simulink model "Simscape_crane_software_model"  (R2016b)
settings: Solver=ode15s  StartTime=0.0  StopTime=3  RelTol=1e-3  EnableMultiTasking=on
values from neighbouring files (symbols this model uses):
  m = 0.47    [SSmodelParams.mat]
  MR = 1.71    [SSmodelParams.mat]
  TxBreak = 0    [setup.m]
  TxCoulomb = 2.5    [setup.m]
  TxVisc = 49.1750    (= 49.175)    [setup.m]
  TyBreak = 0    [setup.m]
  TyCoulomb = 1.8    [setup.m]
  xZero = 0    [setup.m]
  yZero = 0    [setup.m]
undefined symbols (not defined in the file or in its folder): sigbuilder_block, TzBreak, TzCoulomb, X, xRange, Y, yRange, Z, zRange, zZero
undefined symbols (not defined in the file): M, TorqueMultX, TorqueMultY, TorqueMultZ, TxTrans, TyTrans, TyVisc, TzTrans, TzVisc
libraries: sm_lib x146, fl_lib x62, nesl_utility x24, elec_lib x9, simulink x6, sm_double_wishbone_suspension_lib x4, aerolibtransform2 x1
(part 11 of 14)

== system Simscape_crane_software_model/0.4 ==
  Demux : Demux  Tag=STV Demux  Outputs=1
  FromWs : FromWorkspace  Tag=STV FromWs  VariableName=tuvar  SampleTime=0
      SigBuilderData=|
      | common.afterFinalStr = 'Extrapolate'
      | common.sampleTime = 0
      | dataSet.timeRange = [0 10]
      | dataSet.name = 'Group 1'
      | sbobj.Groups.Name = 'Group 1'
      | sbobj.Groups.Signals.Name = 'Signal 1'
      | sbobj.Groups.Signals.XData = [0 1 1 2 2 10]
      | sbobj.Groups.Signals.YData = [0 0 0.4 0.4 0 0]
  Signal 1 : Outport  Tag=STV Outport
  wires:
  Demux/1 -> Signal 1/1
  FromWs/1 -> Demux/1

== system Simscape_crane_software_model/0.8 ==
  Demux : Demux  Tag=STV Demux  Outputs=1
  FromWs : FromWorkspace  Tag=STV FromWs  VariableName=tuvar  SampleTime=0
      SigBuilderData=|
      | common.afterFinalStr = 'Extrapolate'
      | common.sampleTime = 0
      | dataSet.timeRange = [0 10]
      | dataSet.name = 'Group 1'
      | sbobj.Groups.Name = 'Group 1'
      | sbobj.Groups.Signals.Name = 'Signal 1'
      | sbobj.Groups.Signals.XData = [0 1 1 2 2 10]
      | sbobj.Groups.Signals.YData = [0 0 0.8 0.8 0 0]
  Signal 1 : Outport  Tag=STV Outport
  wires:
  FromWs/1 -> Demux/1
  Demux/1 -> Signal 1/1

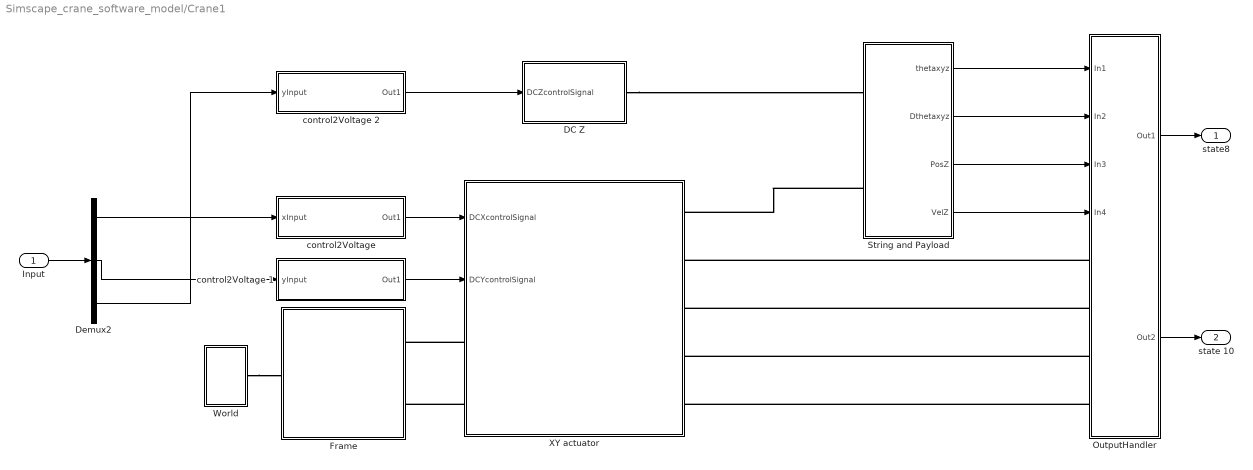
== system Simscape_crane_software_model/Crane1 ==
  Input : Inport
  DC Z : Subsystem
  Demux2 : Demux  Outputs=3
  Frame : Subsystem
  OutputHandler : Subsystem
  String and Payload : Subsystem
  World : Subsystem
  XY actuator : Subsystem
  "control2Voltage " : Subsystem
      mask Display:
      | port_label('output', 1, 'pwm_out')
      | port_label('input', 1, 'controlVal')
  control2Voltage 1 : Subsystem
      mask Display:
      | port_label('output', 1, 'pwm_out')
      | port_label('input', 1, 'controlVal')
  control2Voltage 2 : Subsystem
      mask Display:
      | port_label('output', 1, 'pwm_out')
      | port_label('input', 1, 'controlVal')
  "state8 " : Outport
  state 10 : Outport  Port=2
  wires:
  "control2Voltage "/1(Out1) -> XY actuator/1(DCXcontrolSignal)
  control2Voltage 1/1(Out1) -> XY actuator/2(DCYcontrolSignal)
  Demux2/1 -> "control2Voltage "/1(xInput)
  Demux2/2 -> control2Voltage 1/1(yInput)
  Input/1 -> Demux2/1
  Demux2/3 -> control2Voltage 2/1(yInput)
  control2Voltage 2/1(Out1) -> DC Z/1(DCZcontrolSignal)
  String and Payload/1(thetaxyz) -> OutputHandler/1(In1)
  String and Payload/2(Dthetaxyz) -> OutputHandler/2(In2)
  String and Payload/3("PosZ ") -> OutputHandler/3(In3)
  String and Payload/4(VelZ) -> OutputHandler/4(In4)
  OutputHandler/1(Out1) -> "state8 "/1
  OutputHandler/2(Out2) -> state 10/1
  connections:
  World/RConn1 -- Frame/LConn1
  XY actuator/LConn1 -- Frame/RConn1
  XY actuator/LConn2 -- Frame/RConn2
  String and Payload/LConn2 -- XY actuator/RConn1
  DC Z/RConn1 -- String and Payload/LConn1
  OutputHandler/LConn1 -- XY actuator/RConn2
  OutputHandler/LConn2 -- XY actuator/RConn3
  OutputHandler/LConn3 -- XY actuator/RConn4
  OutputHandler/LConn4 -- XY actuator/RConn5

== system Simscape_crane_software_model/Crane1/DC Z ==
  DCZcontrolSignal : Inport
  " Lead Screw" : fl_lib/Mechanical/Mechanisms/Wheel and Axle  R=6 cm  or=1  t_specify=off  t_priority=High  t=0 N*m  f_specify=off  f_priority=High  f=0 N
  DC Motor2 : elec_lib/Actuators & Drivers/Rotational Actuators/DC Motor  parameterization=2  Ra=3.9 Ohm  La=1.2e-5 H  emf_or_torque=1  Kv=7.2e-5 V/rpm  Ki=6.876e-4 N*m/A  T_stall=10000 mN*m  w_max=190 rpm  w_rated=190 rpm  P_rated=0.08 W  V_rated=24 V  J=0.01 g*cm^2  lam_param=1  lam=0 N*m/(rad/s)  i_noload=0 A  V_i_noload=1.5 V  speed0=0 rpm  alpha=0.00393 1/K  Tmeas=25 C  thermal_mass=100 J/K  initial_temperature=25 C
  Force Sensor : fl_lib/Mechanical/Mechanical Sensors/Ideal Force Sensor
  Gear Box : fl_lib/Mechanical/Mechanisms/Gear Box  Tag=Factory Generic  ratio=1/30  t_in_specify=off  t_in_priority=High  t_in=0 N*m  t_out_specify=off  t_out_priority=High  t_out=0 N*m
  Mechanical Rotational Reference1 : fl_lib/Mechanical/Rotational Elements/Mechanical Rotational Reference
  Mechanical Translational Reference4 : fl_lib/Mechanical/Translational Elements/Mechanical Translational Reference
  PS Gain : fl_lib/Physical Signals/Functions/PS Gain  gain=-Uz
  PWM & H-Bridge1 : Subsystem
  SL2V_1 : Subsystem
  Conn1 : PMIOPort  Port=1  Side=Right
  wires:
  DCZcontrolSignal/1 -> SL2V_1/1(SL)
  connections:
  Force Sensor/RConn2 -- PS Gain/LConn1
  Mechanical Translational Reference4/LConn1 -- Force Sensor/LConn1
  Mechanical Rotational Reference1/LConn1 -- DC Motor2/RConn2
  Gear Box/RConn1 -- " Lead Screw"/LConn1
  Force Sensor/RConn1 -- " Lead Screw"/RConn1
  DC Motor2/LConn2 -- Gear Box/LConn1
  PWM & H-Bridge1/RConn2 -- DC Motor2/RConn1
  SL2V_1/RConn2 -- PWM & H-Bridge1/LConn2
  SL2V_1/RConn3 -- PWM & H-Bridge1/LConn3
  SL2V_1/RConn4 -- PWM & H-Bridge1/LConn4
  SL2V_1/RConn1 -- PWM & H-Bridge1/LConn1
  PWM & H-Bridge1/RConn1 -- DC Motor2/LConn1
  Conn1/RConn1 -- PS Gain/RConn1

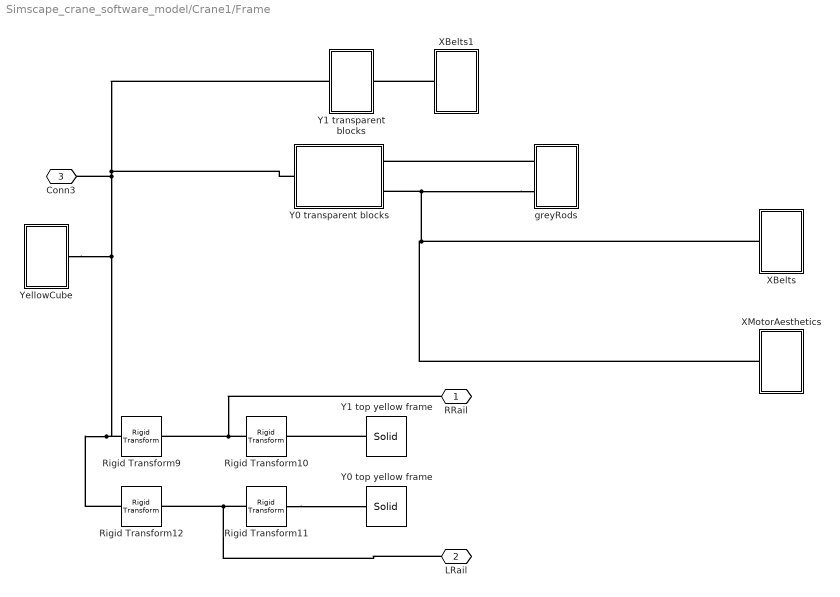
== system Simscape_crane_software_model/Crane1/Frame ==
  Rigid Transform10 : sm_lib/Frames and Transforms/Rigid Transform  TranslationMethod=None  TranslationStandardOffset=0  TranslationLengthUnit=m  TranslationStandardAxis=+Z  TranslationCartesianOffset="[-0.5 1  0]"  TranslationROffset=0  TranslationROffsetUnits=m  TranslationZOffset=0  TranslationZOffsetUnits=m  TranslationThetaOffset=0  TranslationThetaOffsetUnits=deg  RotationMethod=StandardAxis  RotationAngleUnits=deg  RotationStandardAxis=+Y  RotationAngle=90  RotationArbitraryAxis=[0 0 1]  FollAlignAxisA=+X  BaseAlignAxisA=+Y  FollAlignAxisB=+Y  BaseAlignAxisB=+Z  RotationSequenceAxes=FollowerAxes  RotationSequence=XYX  RotationSequenceAngles=[0 0 0]  RotationSequenceAnglesUnits=deg  RotationMatrix=[1 0 0; 0 1 0; 0 0 1]
  Rigid Transform11 : sm_lib/Frames and Transforms/Rigid Transform  TranslationMethod=None  TranslationStandardOffset=0  TranslationLengthUnit=m  TranslationStandardAxis=+Z  TranslationCartesianOffset="[-0.5 1  0]"  TranslationROffset=0  TranslationROffsetUnits=m  TranslationZOffset=0  TranslationZOffsetUnits=m  TranslationThetaOffset=0  TranslationThetaOffsetUnits=deg  RotationMethod=StandardAxis  RotationAngleUnits=deg  RotationStandardAxis=+Y  RotationAngle=90  RotationArbitraryAxis=[0 0 1]  FollAlignAxisA=+X  BaseAlignAxisA=+Y  FollAlignAxisB=+Y  BaseAlignAxisB=+Z  RotationSequenceAxes=FollowerAxes  RotationSequence=XYX  RotationSequenceAngles=[0 0 0]  RotationSequenceAnglesUnits=deg  RotationMatrix=[1 0 0; 0 1 0; 0 0 1]
  Rigid Transform12 : sm_lib/Frames and Transforms/Rigid Transform  TranslationMethod=Cartesian  TranslationStandardOffset=0  TranslationLengthUnit=m  TranslationStandardAxis=+Z  TranslationCartesianOffset=[0 -0.5 1]  TranslationROffset=0  TranslationROffsetUnits=m  TranslationZOffset=0  TranslationZOffsetUnits=m  TranslationThetaOffset=0  TranslationThetaOffsetUnits=deg  RotationMethod=None  RotationAngleUnits=deg  RotationStandardAxis=+X  RotationAngle=90  RotationArbitraryAxis=[0 0 1]  FollAlignAxisA=+X  BaseAlignAxisA=+Y  FollAlignAxisB=+Y  BaseAlignAxisB=+Z  RotationSequenceAxes=FollowerAxes  RotationSequence=XYX  RotationSequenceAngles=[0 0 0]  RotationSequenceAnglesUnits=deg  RotationMatrix=[1 0 0; 0 1 0; 0 0 1]
  Rigid Transform9 : sm_lib/Frames and Transforms/Rigid Transform  TranslationMethod=Cartesian  TranslationStandardOffset=0  TranslationLengthUnit=m  TranslationStandardAxis=+Z  TranslationCartesianOffset=[0 0.5 1]  TranslationROffset=0  TranslationROffsetUnits=m  TranslationZOffset=0  TranslationZOffsetUnits=m  TranslationThetaOffset=0  TranslationThetaOffsetUnits=deg  RotationMethod=None  RotationAngleUnits=deg  RotationStandardAxis=+X  RotationAngle=90  RotationArbitraryAxis=[0 0 1]  FollAlignAxisA=+X  BaseAlignAxisA=+Y  FollAlignAxisB=+Y  BaseAlignAxisB=+Z  RotationSequenceAxes=FollowerAxes  RotationSequence=XYX  RotationSequenceAngles=[0 0 0]  RotationSequenceAnglesUnits=deg  RotationMatrix=[1 0 0; 0 1 0; 0 0 1]
  XBelts : Subsystem
  XBelts1 : Subsystem
  XMotorAesthetics : Subsystem
  Y0 top yellow frame : sm_lib/Body Elements/Solid  InertiaType=CalculateFromGeometry  Mass=1  MassUnits=kg  CenterOfMass=[0 0 0]  CenterOfMassUnits=m  MomentsOfInertia=[1 1 1]  MomentsOfInertiaUnits=kg*m^2  ProductsOfInertia=[0 0 0]  ProductsOfInertiaUnits=kg*m^2  DensityBased=on  Density=1000  DensityUnits=kg/(m^3)  DoExposeReferenceFrame=on  SerializedFrames=<Frames/>  GraphicType=FromGeometry  MarkerShape=Sphere  MarkerSize=10  MarkerSizeUnits=m  GraphicVisPropType=SimpleVisualProperties  GraphicDiffuseColor=[1.0 1.0 0.2]  GraphicSpecularColor=[0.5 0.5 0.5 1.0]  GraphicAmbientColor=[0.15 0.15 0.15 1.0]  GraphicEmissiveColor=[0.0 0.0 0.0 1.0]  GraphicShininess=75  GraphicOpacity=1.0  GeometryShape=Brick  RectangleSize=[1 1]  RectangleSizeUnits=m  BrickDimensions=[0.04 0.04 1.04]  BrickDimensionUnits=m  CylinderRadius=0.02  CylinderRadiusUnits=m  CylinderLength=1  CylinderLengthUnits=m  SphereRadius=1  SphereRadiusUnits=m  EllipsoidRadii=[1 1 1]  EllipsoidRadiiUnits=m  ExtrusionCrossSection=[1 1; -1 1; -1 -1; 1 -1]  ExtrusionCrossSectionUnits=m  ExtrusionLength=1  ExtrusionLengthUnits=m  PolygonNumSides=3  PolygonOuterRadius=1  PolygonOuterRadiusUnits=m  ExtGeomFileType=STL  ExtGeomFileUnits=m  RevolutionCrossSection=[1 1; 1 -1; 2 -1; 2 1]  RevolutionCrossSectionUnits=m  RevolutionExtent=Full  RevolutionAngle=180  RevolutionAngleUnits=deg
  Y0 transparent blocks : Subsystem
  Y1 top yellow frame : sm_lib/Body Elements/Solid  InertiaType=CalculateFromGeometry  Mass=1  MassUnits=kg  CenterOfMass=[0 0 0]  CenterOfMassUnits=m  MomentsOfInertia=[1 1 1]  MomentsOfInertiaUnits=kg*m^2  ProductsOfInertia=[0 0 0]  ProductsOfInertiaUnits=kg*m^2  DensityBased=on  Density=1000  DensityUnits=kg/(m^3)  DoExposeReferenceFrame=on  SerializedFrames=<Frames/>  GraphicType=FromGeometry  MarkerShape=Sphere  MarkerSize=10  MarkerSizeUnits=m  GraphicVisPropType=SimpleVisualProperties  GraphicDiffuseColor=[1.0 1.0 0.2]  GraphicSpecularColor=[0.5 0.5 0.5 1.0]  GraphicAmbientColor=[0.15 0.15 0.15 1.0]  GraphicEmissiveColor=[0.0 0.0 0.0 1.0]  GraphicShininess=75  GraphicOpacity=1.0  GeometryShape=Brick  RectangleSize=[1 1]  RectangleSizeUnits=m  BrickDimensions=[0.04 0.04 1.04]  BrickDimensionUnits=m  CylinderRadius=0.02  CylinderRadiusUnits=m  CylinderLength=1  CylinderLengthUnits=m  SphereRadius=1  SphereRadiusUnits=m  EllipsoidRadii=[1 1 1]  EllipsoidRadiiUnits=m  ExtrusionCrossSection=[1 1; -1 1; -1 -1; 1 -1]  ExtrusionCrossSectionUnits=m  ExtrusionLength=1  ExtrusionLengthUnits=m  PolygonNumSides=3  PolygonOuterRadius=1  PolygonOuterRadiusUnits=m  ExtGeomFileType=STL  ExtGeomFileUnits=m  RevolutionCrossSection=[1 1; 1 -1; 2 -1; 2 1]  RevolutionCrossSectionUnits=m  RevolutionExtent=Full  RevolutionAngle=180  RevolutionAngleUnits=deg
  Y1 transparent blocks : Subsystem
  YellowCube : Subsystem
  greyRods : Subsystem
  RRail : PMIOPort  Port=1  Side=Right
  LRail : PMIOPort  Port=2  Side=Right
  Conn3 : PMIOPort  Port=3  Side=Left
  connections:
  Rigid Transform10/LConn1 -- RRail/RConn1 -- Rigid Transform9/RConn1
  Rigid Transform11/LConn1 -- LRail/RConn1 -- Rigid Transform12/RConn1
  Y1 top yellow frame/RConn1 -- Rigid Transform10/RConn1
  Rigid Transform11/RConn1 -- Y0 top yellow frame/RConn1
  YellowCube/RConn1 -- Rigid Transform12/LConn1 -- Rigid Transform9/LConn1 -- Y1 transparent blocks/LConn1 -- Y0 transparent blocks/LConn1 -- Conn3/RConn1
  greyRods/LConn2 -- XMotorAesthetics/LConn1 -- XBelts/RConn1 -- Y0 transparent blocks/RConn2
  greyRods/LConn1 -- Y0 transparent blocks/RConn1
  XBelts1/RConn1 -- Y1 transparent blocks/RConn1

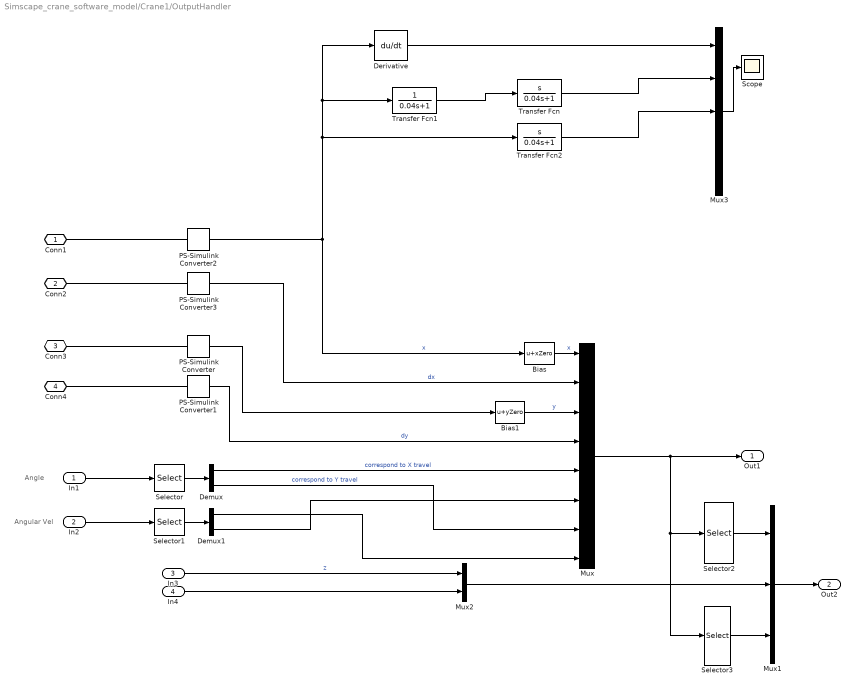
== system Simscape_crane_software_model/Crane1/OutputHandler ==
  note: Angular Vel
  note: Angle
  In1 : Inport
  In2 : Inport  Port=2
  In3 : Inport  Port=3
  In4 : Inport  Port=4
  Bias : Bias  Bias=xZero
  Bias1 : Bias  Bias=yZero
  Demux : Demux  Outputs=2
  Demux1 : Demux  Outputs=2
  Derivative : Derivative
  Mux : Mux  Inputs=8
  Mux1 : Mux  Inputs=3
  Mux2 : Mux  Inputs=2
  Mux3 : Mux  Inputs=5
  PS-Simulink Converter{,1..3} (4 alike) : nesl_utility/PS-Simulink Converter  PhysicalDomain=network_engine_domain  SubClassName=ps_output  LeftPortType=input  RightPortType=output  PseudoPeriodic=off  Frequencies=[]  Unit=1  AffineConversion=off
  Scope : Scope
  Selector : Selector  InputPortWidth=3  IndexOptions=Index vector (dialog)  Indices=[2 3]  OutputSizes=1
  Selector1 : Selector  InputPortWidth=3  IndexOptions=Index vector (dialog)  Indices=[1 2]  OutputSizes=1
  Selector2 : Selector  InputPortWidth=8  IndexOptions=Index vector (dialog)  Indices=1:4  OutputSizes=1
  Selector3 : Selector  InputPortWidth=8  IndexOptions=Index vector (dialog)  Indices=5:8  OutputSizes=1
  Transfer Fcn : TransferFcn  Numerator=[1 0]  Denominator=[0.04 1]
  Transfer Fcn1 : TransferFcn  Numerator=[0 1]  Denominator=[0.04 1]
  Transfer Fcn2 : TransferFcn  Numerator=[1 0]  Denominator=[0.04 1]
  Conn1 : PMIOPort  Port=1  Side=Left
  Conn2 : PMIOPort  Port=2  Side=Left
  Conn3 : PMIOPort  Port=3  Side=Left
  Conn4 : PMIOPort  Port=4  Side=Left
  Out1 : Outport
  Out2 : Outport  Port=2
  wires:
  In1/1 -> Selector/1
  Demux/2 -> Mux/7  "correspond to Y travel"
  Selector/1 -> Demux/1
  Demux/1 -> Mux/5  "correspond to X travel"
  Demux1/2 -> Mux/6
  Selector1/1 -> Demux1/1
  Demux1/1 -> Mux/8
  In2/1 -> Selector1/1
  Mux/1 -> Out1/1, Selector3/1, Selector2/1
  PS-Simulink Converter2/1 -> Transfer Fcn2/1, Derivative/1, Transfer Fcn1/1, Bias/1  "x"
  PS-Simulink Converter3/1 -> Mux/2  "dx"
  PS-Simulink Converter/1 -> Bias1/1
  PS-Simulink Converter1/1 -> Mux/4  "dy"
  Bias/1 -> Mux/1  "x"
  Bias1/1 -> Mux/3  "y"
  In4/1 -> Mux2/2
  In3/1 -> Mux2/1  "z"
  Selector2/1 -> Mux1/1
  Mux2/1 -> Mux1/2
  Selector3/1 -> Mux1/3
  Mux1/1 -> Out2/1
  Transfer Fcn/1 -> Mux3/2
  Derivative/1 -> Mux3/1
  Mux3/1 -> Scope/1
  Transfer Fcn1/1 -> Transfer Fcn/1
  Transfer Fcn2/1 -> Mux3/3
  connections:
  PS-Simulink Converter/LConn1 -- Conn3/RConn1
  PS-Simulink Converter2/LConn1 -- Conn1/RConn1
  PS-Simulink Converter1/LConn1 -- Conn4/RConn1
  PS-Simulink Converter3/LConn1 -- Conn2/RConn1

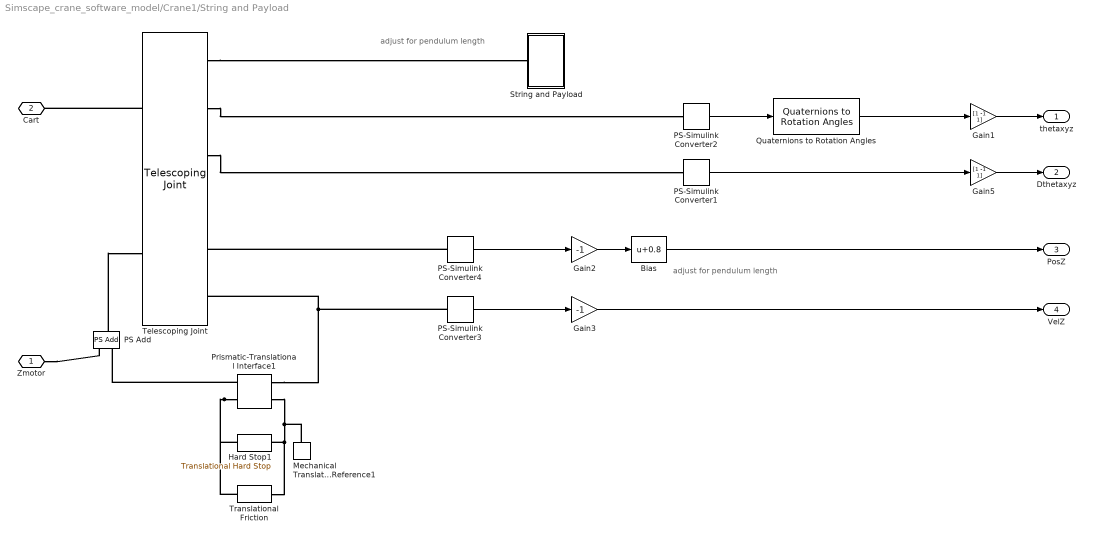
== system Simscape_crane_software_model/Crane1/String and Payload ==
  note: adjust for pendulum length
  note: adjust for pendulum length
  Bias : Bias  Bias=0.8
  Gain1 : Gain  Gain=[1 -1 1]
  Gain2 : Gain  Gain=-1
  Gain3 : Gain  Gain=-1
  Gain5 : Gain  Gain=[1 -1 1]
  Hard Stop1 : fl_lib/Mechanical/Translational Elements/Translational Hard Stop  upper_bnd=zZero-zRange(1) m  lower_bnd=-(zRange(2)-zZero) m  stiff_up=2e6 N/m  stiff_low=2e6 N/m  D_up=1000 N/(m/s)  D_low=1000 N/(m/s)  v_specify=off  v_priority=High  v=0 m/s  f_specify=off  f_priority=High  f=0 N  x_specify=off  x_priority=High  x=1 cm
  Mechanical Translational Reference1 : fl_lib/Mechanical/Translational Elements/Mechanical Translational Reference
  PS Add : fl_lib/Physical Signals/Functions/PS Add
  PS-Simulink Converter{1..4} (4 alike) : nesl_utility/PS-Simulink Converter  PhysicalDomain=network_engine_domain  SubClassName=ps_output  LeftPortType=input  RightPortType=output  PseudoPeriodic=off  Frequencies=[]  Unit=1  AffineConversion=off
  Prismatic-Translational Interface1 : sm_double_wishbone_suspension_lib/Testing Platform/Prismatic-Translational Interface
  Quaternions to Rotation Angles : aerolibtransform2/Quaternions to Rotation Angles  rotationOrder=ZYX
  "String and Payload " : Subsystem
  Telescoping Joint : sm_lib/Joints/Telescoping Joint  SenseConstraintForce=off  SenseConstraintForceX=off  SenseConstraintForceY=off  SenseConstraintForceZ=off  SenseConstraintTorque=off  SenseConstraintTorqueX=off  SenseConstraintTorqueY=off  SenseConstraintTorqueZ=off  SenseTotalForce=off  SenseTotalForceX=off  SenseTotalForceY=off  SenseTotalForceZ=off  SenseTotalTorque=off  SenseTotalTorqueX=off  SenseTotalTorqueY=off  SenseTotalTorqueZ=off  CompositeWrenchDir=FollowerOnBase  CompositeWrenchFrame=BaseFrame  SphDefPosRotationMethod=None  SphDefPosRotationAngleUnits=deg  SphDefPosRotationStandardAxis=+Z  SphDefPosRotationAngle=0.0  SphDefPosRotationArbitraryAxis=[0 0 1]  SphDefPosFollAlignAxisA=+X  SphDefPosBaseAlignAxisA=+Y  SphDefPosFollAlignAxisB=+Y  SphDefPosBaseAlignAxisB=+Z  SphDefPosRotationSequenceAxes=FollowerAxes  SphDefPosRotationSequence=XYX  SphDefPosRotationSequenceAngles=[0 0 0]  SphDefPosRotationSequenceAnglesUnits=deg  SphDefPosRotationMatrix=[1 0 0; 0 1 0; 0 0 1]  SphEqPosRotationMethod=None  SphEqPosRotationAngleUnits=deg  SphEqPosRotationStandardAxis=+Z  SphEqPosRotationAngle=0.0  SphEqPosRotationArbitraryAxis=[0 0 1]  SphEqPosFollAlignAxisA=+X  SphEqPosBaseAlignAxisA=+Y  SphEqPosFollAlignAxisB=+Y  SphEqPosBaseAlignAxisB=+Z  SphEqPosRotationSequenceAxes=FollowerAxes  SphEqPosRotationSequence=XYX  SphEqPosRotationSequenceAngles=[0 0 0]  SphEqPosRotationSequenceAnglesUnits=deg  SphEqPosRotationMatrix=[1 0 0; 0 1 0; 0 0 1]  SphSpringStiffness=0  SphSpringStiffnessUnits=N*m/deg  SphDampingCoefficient=0.0025  SphDampingCoefficientUnits=N*m/(rad/s)  SphActuateTorqueX=off  SphActuateTorqueY=off  SphActuateTorqueZ=off  SphActuateTorque=off  SphTorqueActuationMode=NoTorque  SphMotionActuationMode=ComputedMotion  SphActuationFrame=BaseFrame  SphSensePosition=on  SphSenseVelocityX=off  SphSenseVelocityY=off  SphSenseVelocityZ=off  SphSenseVelocity=on  SphSenseAccelerationX=off  SphSenseAccelerationY=off  SphSenseAccelerationZ=off  SphSenseAcceleration=on  SphSenseTorqueX=off  SphSenseTorqueY=off  SphSenseTorqueZ=off  SphSenseTorqueForce=off  SphSensingFrame=BaseFrame  SphPositionTargetRotationMethod=None  SphPositionTargetRotationAngleUnits=deg  SphPositionTargetRotationStandardAxis=+Z  SphPositionTargetRotationAngle=0.0  SphPositionTargetRotationArbitraryAxis=[0 0 1]  SphPositionTargetFollAlignAxisA=+X  SphPositionTargetBaseAlignAxisA=+Y  SphPositionTargetFollAlignAxisB=+Y  SphPositionTargetBaseAlignAxisB=+Z  SphPositionTargetRotationSequenceAxes=FollowerAxes  SphPositionTargetRotationSequence=XYX  SphPositionTargetRotationSequenceAngles=[0 0 0]  SphPositionTargetRotationSequenceAnglesUnits=deg  SphPositionTargetRotationMatrix=[1 0 0; 0 1 0; 0 0 1]  SphPositionTargetSpecify=off  SphPositionTargetPriority=High  SphVelocityTargetValue=[0 0 0]  SphVelocityTargetValueUnits=deg/s  SphVelocityTargetSpecify=off  SphVelocityTargetPriority=High  SphVelocityTargetInFollowerFrame=on  PzEquilibriumPosition=0  PzEquilibriumPositionUnits=m  PzSpringStiffness=0  PzSpringStiffnessUnits=N/m  PzDampingCoefficient=0  PzDampingCoefficientUnits=N/(m/s)  PzTorqueActuationMode=InputTorque  PzMotionActuationMode=ComputedMotion  PzSensePosition=on  PzSenseVelocity=on  PzSenseAcceleration=off  PzSenseTorqueForce=off  PzPositionTargetSpecify=off  PzPositionTargetPriority=High  PzPositionTargetValue=0  PzPositionTargetValueUnits=m  PzVelocityTargetSpecify=off  PzVelocityTargetPriority=High  PzVelocityTargetValue=0  PzVelocityTargetValueUnits=m/s
  Translational Friction : fl_lib/Mechanical/Translational Elements/Translational Friction  brkwy_frc=TzBreak+TzCoulomb N  Col_frc=TzCoulomb N  visc_coef=TzVisc N/(m/s)  trans_coef=10 s/m  vel_thr=1e-4 m/s  v_specify=off  v_priority=None  v=0 m/s  f_specify=off  f_priority=None  f=0 N
  Zmotor : PMIOPort  Port=1  Side=Left
  Cart : PMIOPort  Port=2  Side=Left
  thetaxyz : Outport
  Dthetaxyz : Outport  Port=2
  "PosZ " : Outport  Port=3
  VelZ : Outport  Port=4
  wires:
  PS-Simulink Converter2/1 -> Quaternions to Rotation Angles/1
  Quaternions to Rotation Angles/1 -> Gain1/1
  PS-Simulink Converter1/1 -> Gain5/1
  Gain1/1 -> thetaxyz/1
  Gain5/1 -> Dthetaxyz/1
  PS-Simulink Converter3/1 -> Gain3/1
  PS-Simulink Converter4/1 -> Gain2/1
  Bias/1 -> "PosZ "/1
  Gain2/1 -> Bias/1
  Gain3/1 -> VelZ/1
  connections:
  Telescoping Joint/LConn1 -- Cart/RConn1
  Telescoping Joint/RConn2 -- PS-Simulink Converter2/LConn1
  Telescoping Joint/RConn3 -- PS-Simulink Converter1/LConn1
  Telescoping Joint/RConn1 -- "String and Payload "/LConn1
  Prismatic-Translational Interface1/RConn2 -- Hard Stop1/RConn1 -- Translational Friction/RConn1
  Mechanical Translational Reference1/LConn1 -- Prismatic-Translational Interface1/LConn2 -- Translational Friction/LConn1 -- Hard Stop1/LConn1
  Prismatic-Translational Interface1/RConn1 -- PS Add/LConn2
  Zmotor/RConn1 -- PS Add/LConn1
  Prismatic-Translational Interface1/LConn1 -- Telescoping Joint/RConn6 -- PS-Simulink Converter3/LConn1
  PS Add/RConn1 -- Telescoping Joint/LConn2
  PS-Simulink Converter4/LConn1 -- Telescoping Joint/RConn5

== system Simscape_crane_software_model/Crane1/World ==
  Mechanism Configuration : sm_lib/Utilities/Mechanism Configuration  UniformGravity=Constant  GravityVector=[0 0 -9.81]  GravityUnits=m/s^2  LinearizationDelta=0.001
  Solver Configuration : nesl_utility/Solver Configuration  PhysicalDomain=network_engine_domain  SubClassName=solver  LeftPortType=input  RightPortType=generic  Accelerate=off  Tones=[]  Harmonics=[]  SimulateNoise=off  Profile=off  UseLocalSampling=off  EnableSwitchedLinearOptims=on  FrequencyDomain=off  UseCCode=off  RelTol=0.001  AbsTol=1e-06  MinStep=1e-09  ToWorkspace=off  RevertToSquareIcSolve=off  NumHomotopyIterations=100  PhasorMode=off  PhasorModeNumHarmonics=1  OverrideAbsTol=off  DoDC=off  ResidualTolerance=1e-09  UseLocalSolver=off  LocalSolverChoice=NE_TRAPEZOIDAL_ADVANCER  LocalSolverSampleTime=0.001  DoFixedCost=off  MaxNonlinIter=3  MaxModeIter=2  LinearAlgebra=Sparse  DelaysMemoryBudget=1024  AutomaticFiltering=on  FilteringTimeConstant=0.001
  World Frame : sm_lib/Frames and Transforms/World Frame
  base : sm_lib/Body Elements/Solid  InertiaType=PointMass  Mass=6e24  MassUnits=kg  CenterOfMass=[0 0 0]  CenterOfMassUnits=m  MomentsOfInertia=[1 1 1]  MomentsOfInertiaUnits=kg*m^2  ProductsOfInertia=[0 0 0]  ProductsOfInertiaUnits=kg*m^2  DensityBased=off  Density=1000  DensityUnits=kg/(m^3)  DoExposeReferenceFrame=on  SerializedFrames=<Frames/>  GraphicType=FromGeometry  MarkerShape=Sphere  MarkerSize=10  MarkerSizeUnits=m  GraphicVisPropType=SimpleVisualProperties  GraphicDiffuseColor=[0.5 0.5 0.5]  GraphicSpecularColor=[0.5 0.5 0.5 1.0]  GraphicAmbientColor=[0.15 0.15 0.15 1.0]  GraphicEmissiveColor=[0.0 0.0 0.0 1.0]  GraphicShininess=75  GraphicOpacity=1.0  GeometryShape=Brick  RectangleSize=[1 1]  RectangleSizeUnits=m  BrickDimensions=[1 1 0.01]  BrickDimensionUnits=m  CylinderRadius=0.02  CylinderRadiusUnits=m  CylinderLength=1  CylinderLengthUnits=m  SphereRadius=1  SphereRadiusUnits=m  EllipsoidRadii=[1 1 1]  EllipsoidRadiiUnits=m  ExtrusionCrossSection=[1 1; -1 1; -1 -1; 1 -1]  ExtrusionCrossSectionUnits=m  ExtrusionLength=1  ExtrusionLengthUnits=m  PolygonNumSides=3  PolygonOuterRadius=1  PolygonOuterRadiusUnits=m  ExtGeomFileType=STL  ExtGeomFileUnits=m  RevolutionCrossSection=[1 1; 1 -1; 2 -1; 2 1]  RevolutionCrossSectionUnits=m  RevolutionExtent=Full  RevolutionAngle=180  RevolutionAngleUnits=deg
  Conn1 : PMIOPort  Port=1  Side=Right
  connections:
  World Frame/RConn1 -- base/RConn1 -- Conn1/RConn1 -- Solver Configuration/RConn1 -- Mechanism Configuration/RConn1

== system Simscape_crane_software_model/Crane1/XY actuator ==
  DCXcontrolSignal : Inport
  DCYcontrolSignal : Inport  Port=2
  DC Y : Subsystem
  X rail : Subsystem
  Y cart : Subsystem
  Conn5 : PMIOPort  Port=1  Side=Right
  XPos : PMIOPort  Port=2  Side=Right
  XVel : PMIOPort  Port=3  Side=Right
  YPos : PMIOPort  Port=4  Side=Right
  "YVel " : PMIOPort  Port=5  Side=Right
  RRail : PMIOPort  Port=6  Side=Left
  LRail : PMIOPort  Port=7  Side=Left
  wires:
  DCYcontrolSignal/1 -> DC Y/1(DCYcontrolSignal)
  DCXcontrolSignal/1 -> X rail/1(DCXcontrolSignal1)
  connections:
  X rail/RConn1 -- XPos/RConn1
  X rail/LConn1 -- RRail/RConn1
  X rail/LConn2 -- LRail/RConn1
  Y cart/RConn1 -- YPos/RConn1
  Conn5/RConn1 -- Y cart/RConn2
  X rail/RConn2 -- Y cart/LConn1
  XVel/RConn1 -- X rail/RConn3
  "YVel "/RConn1 -- Y cart/RConn3
  DC Y/RConn1 -- Y cart/LConn2

== system Simscape_crane_software_model/Crane1/control2Voltage  ==
  note: Force applied on the cart at 100% motor torque is 12.9 N
  xInput : Inport
  Abs2 : Abs
  Compare To Zero3 : simulink/Logic and Bit Operations/Compare To Zero  relop===  OutDataTypeStr=boolean
  Compare To Zero4 : simulink/Logic and Bit Operations/Compare To Zero  relop=<  OutDataTypeStr=boolean
  Data Type Conversion2 : DataTypeConversion  OutDataTypeStr=double
  Data Type Conversion3 : DataTypeConversion  OutDataTypeStr=double
  Mux2 : Mux  Inputs=3
  Saturation : Saturate  UpperLimit=1  LowerLimit=-1
  Out1 : Outport
  wires:
  Compare To Zero3/1 -> Data Type Conversion2/1
  Data Type Conversion3/1 -> Mux2/2
  Compare To Zero4/1 -> Data Type Conversion3/1
  Mux2/1 -> Out1/1
  xInput/1 -> Compare To Zero4/1, Abs2/1, Compare To Zero3/1  "xInput"
  Data Type Conversion2/1 -> Mux2/3
  Abs2/1 -> Saturation/1
  Saturation/1 -> Mux2/1

== system Simscape_crane_software_model/Crane1/control2Voltage 1 ==
  yInput : Inport
  Abs2 : Abs
  Compare To Zero3 : simulink/Logic and Bit Operations/Compare To Zero  relop===  OutDataTypeStr=boolean
  Compare To Zero4 : simulink/Logic and Bit Operations/Compare To Zero  relop=<  OutDataTypeStr=boolean
  Data Type Conversion2 : DataTypeConversion  OutDataTypeStr=double
  Data Type Conversion3 : DataTypeConversion  OutDataTypeStr=double
  Mux2 : Mux  Inputs=3
  Saturation : Saturate  UpperLimit=1  LowerLimit=-1
  Out1 : Outport
  wires:
  Saturation/1 -> Mux2/1
  Abs2/1 -> Saturation/1
  Data Type Conversion2/1 -> Mux2/3
  yInput/1 -> Compare To Zero3/1, Abs2/1, Compare To Zero4/1  "yInput"
  Mux2/1 -> Out1/1
  Compare To Zero4/1 -> Data Type Conversion3/1
  Data Type Conversion3/1 -> Mux2/2
  Compare To Zero3/1 -> Data Type Conversion2/1

== system Simscape_crane_software_model/Crane1/control2Voltage 2 ==
  yInput : Inport
  Abs2 : Abs
  Compare To Zero3 : simulink/Logic and Bit Operations/Compare To Zero  relop===  OutDataTypeStr=boolean
  Compare To Zero4 : simulink/Logic and Bit Operations/Compare To Zero  relop=<  OutDataTypeStr=boolean
  Data Type Conversion2 : DataTypeConversion  OutDataTypeStr=double
  Data Type Conversion3 : DataTypeConversion  OutDataTypeStr=double
  Mux2 : Mux  Inputs=3
  Saturation : Saturate  UpperLimit=1  LowerLimit=-1
  Out1 : Outport
  wires:
  Compare To Zero3/1 -> Data Type Conversion2/1
  Data Type Conversion3/1 -> Mux2/2
  Compare To Zero4/1 -> Data Type Conversion3/1
  Mux2/1 -> Out1/1
  yInput/1 -> Compare To Zero4/1, Abs2/1, Compare To Zero3/1  "yInput"
  Data Type Conversion2/1 -> Mux2/3
  Abs2/1 -> Saturation/1
  Saturation/1 -> Mux2/1

== system Simscape_crane_software_model/Crane1/DC Z/PWM & H-Bridge1 ==
  note: For validation purposes the simulation mode
      | can be set to PWM in both the Controlled PWM
      | and H-Bridge blocks.
  Controlled PWM Voltage : elec_lib/Actuators & Drivers/Drivers/Controlled PWM Voltage  F=10000 Hz  TD=0 s  pulse_width_offset=0 s  Vmin=0 V  Vmax=5 V  Vm=5 V  pwm_or_av=2  event_type=1  sample_time=1e-6 s
  Electrical Reference2 : fl_lib/Electrical/Electrical Elements/Electrical Reference
  H-Bridge : elec_lib/Actuators & Drivers/Drivers/H-Bridge  Venable=2.5 V  Vmax=5 V  Vreverse=2.5 V  Vbrake=2.5 V  Vm=24 V  pwm_or_av=2  discontinuous=0  freewheeling_mode=1  freewheeling_mode_disc=1  Ron=0.1 Ohm  Don=0.1 Ohm  Rload=10 Ohm  Lload=1e-5 H  F=10 kHz  thermal_mass=100 J/K  initial_temperature=298.15 K  Ron2=0.1 Ohm  Don2=0.05 Ohm  Tmeas=298.15 K  Tmeas2=398.15 K
  V+ : PMIOPort  Port=1  Side=Right
  V- : PMIOPort  Port=2  Side=Right
  Vr : PMIOPort  Port=3  Side=Left
  REV : PMIOPort  Port=4  Side=Left
  "brk " : PMIOPort  Port=5  Side=Left
  "gnd " : PMIOPort  Port=6  Side=Left
  connections:
  V+/RConn1 -- H-Bridge/RConn1
  H-Bridge/RConn2 -- V-/RConn1 -- Electrical Reference2/LConn1
  H-Bridge/LConn1 -- Controlled PWM Voltage/RConn1
  Vr/RConn1 -- Controlled PWM Voltage/LConn1
  REV/RConn1 -- H-Bridge/LConn3
  "gnd "/RConn1 -- H-Bridge/LConn2 -- Controlled PWM Voltage/RConn2 -- Controlled PWM Voltage/LConn2
  "brk "/RConn1 -- H-Bridge/LConn4

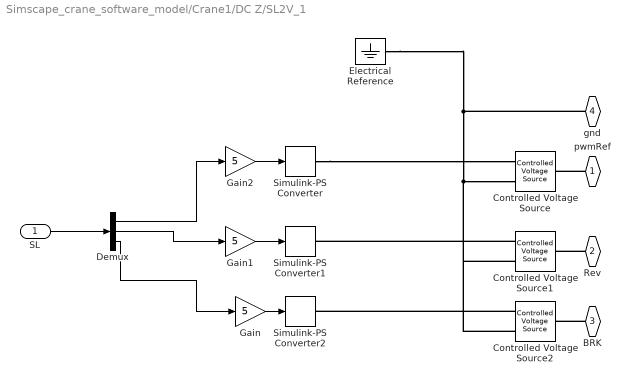
== system Simscape_crane_software_model/Crane1/DC Z/SL2V_1 ==
  SL : Inport
  Controlled Voltage Source : fl_lib/Electrical/Electrical Sources/Controlled Voltage Source
  Controlled Voltage Source1 : fl_lib/Electrical/Electrical Sources/Controlled Voltage Source
  Controlled Voltage Source2 : fl_lib/Electrical/Electrical Sources/Controlled Voltage Source
  Demux : Demux  Outputs=3
  Electrical Reference : fl_lib/Electrical/Electrical Elements/Electrical Reference
  Gain : Gain  Gain=5
  Gain1 : Gain  Gain=5
  Gain2 : Gain  Gain=5
  Simulink-PS Converter : nesl_utility/Simulink-PS Converter  PhysicalDomain=network_engine_domain  SubClassName=ps_input  LeftPortType=input  RightPortType=output  PseudoPeriodic=off  Frequencies=[]  NoiseDistribution=none  NoiseParameters=[]  Unit=V  AffineConversion=off  InputFiltering=off  SimscapeFilterOrder=1  InputFilterTimeConstant=.001  UdotUserProvided=0
  Simulink-PS Converter1 : nesl_utility/Simulink-PS Converter  PhysicalDomain=network_engine_domain  SubClassName=ps_input  LeftPortType=input  RightPortType=output  PseudoPeriodic=off  Frequencies=[]  NoiseDistribution=none  NoiseParameters=[]  Unit=V  AffineConversion=off  InputFiltering=off  SimscapeFilterOrder=1  InputFilterTimeConstant=.001  UdotUserProvided=0
  Simulink-PS Converter2 : nesl_utility/Simulink-PS Converter  PhysicalDomain=network_engine_domain  SubClassName=ps_input  LeftPortType=input  RightPortType=output  PseudoPeriodic=off  Frequencies=[]  NoiseDistribution=none  NoiseParameters=[]  Unit=V  AffineConversion=off  InputFiltering=off  SimscapeFilterOrder=1  InputFilterTimeConstant=.001  UdotUserProvided=0
  pwmRef : PMIOPort  Port=1  Side=Right
  Rev : PMIOPort  Port=2  Side=Right
  BRK : PMIOPort  Port=3  Side=Right
  "gnd " : PMIOPort  Port=4  Side=Right
  wires:
  SL/1 -> Demux/1
  Demux/1 -> Gain2/1
  Demux/3 -> Gain/1
  Gain/1 -> Simulink-PS Converter2/1
  Demux/2 -> Gain1/1
  Gain1/1 -> Simulink-PS Converter1/1
  Gain2/1 -> Simulink-PS Converter/1
  connections:
  Simulink-PS Converter/RConn1 -- Controlled Voltage Source/RConn1
  pwmRef/RConn1 -- Controlled Voltage Source/LConn1
  Electrical Reference/LConn1 -- Controlled Voltage Source/RConn2 -- Controlled Voltage Source1/RConn2 -- Controlled Voltage Source2/RConn2 -- "gnd "/RConn1
  Rev/RConn1 -- Controlled Voltage Source1/LConn1
  Controlled Voltage Source2/RConn1 -- Simulink-PS Converter2/RConn1
  BRK/RConn1 -- Controlled Voltage Source2/LConn1
  Controlled Voltage Source1/RConn1 -- Simulink-PS Converter1/RConn1

== system Simscape_crane_software_model/Crane1/Frame/XBelts ==
  Rigid Transform14 : sm_lib/Frames and Transforms/Rigid Transform  TranslationMethod=StandardAxis  TranslationStandardOffset=0.06  TranslationLengthUnit=m  TranslationStandardAxis=-Z  TranslationCartesianOffset="[-0.5 0  0]"  TranslationROffset=0  TranslationROffsetUnits=m  TranslationZOffset=0  TranslationZOffsetUnits=m  TranslationThetaOffset=0  TranslationThetaOffsetUnits=deg  RotationMethod=None  RotationAngleUnits=deg  RotationStandardAxis=+Y  RotationAngle=90  RotationArbitraryAxis=[0 0 1]  FollAlignAxisA=+X  BaseAlignAxisA=+Y  FollAlignAxisB=+Y  BaseAlignAxisB=+Z  RotationSequenceAxes=FollowerAxes  RotationSequence=XYX  RotationSequenceAngles=[0 0 0]  RotationSequenceAnglesUnits=deg  RotationMatrix=[1 0 0; 0 1 0; 0 0 1]
  Rigid Transform15 : sm_lib/Frames and Transforms/Rigid Transform  TranslationMethod=StandardAxis  TranslationStandardOffset=0.02  TranslationLengthUnit=m  TranslationStandardAxis=+Z  TranslationCartesianOffset="[-0.5 0  0]"  TranslationROffset=0  TranslationROffsetUnits=m  TranslationZOffset=0  TranslationZOffsetUnits=m  TranslationThetaOffset=0  TranslationThetaOffsetUnits=deg  RotationMethod=None  RotationAngleUnits=deg  RotationStandardAxis=+Y  RotationAngle=90  RotationArbitraryAxis=[0 0 1]  FollAlignAxisA=+X  BaseAlignAxisA=+Y  FollAlignAxisB=+Y  BaseAlignAxisB=+Z  RotationSequenceAxes=FollowerAxes  RotationSequence=XYX  RotationSequenceAngles=[0 0 0]  RotationSequenceAnglesUnits=deg  RotationMatrix=[1 0 0; 0 1 0; 0 0 1]
  Rigid Transform19 : sm_lib/Frames and Transforms/Rigid Transform  TranslationMethod=StandardAxis  TranslationStandardOffset=0.43  TranslationLengthUnit=m  TranslationStandardAxis=+X  TranslationCartesianOffset="[-0.5 0  0]"  TranslationROffset=0  TranslationROffsetUnits=m  TranslationZOffset=0  TranslationZOffsetUnits=m  TranslationThetaOffset=0  TranslationThetaOffsetUnits=deg  RotationMethod=None  RotationAngleUnits=deg  RotationStandardAxis=+Y  RotationAngle=90  RotationArbitraryAxis=[0 0 1]  FollAlignAxisA=+X  BaseAlignAxisA=+Y  FollAlignAxisB=+Y  BaseAlignAxisB=+Z  RotationSequenceAxes=FollowerAxes  RotationSequence=XYX  RotationSequenceAngles=[0 0 0]  RotationSequenceAnglesUnits=deg  RotationMatrix=[1 0 0; 0 1 0; 0 0 1]
  belt : sm_lib/Body Elements/Solid  InertiaType=PointMass  Mass=0  MassUnits=kg  CenterOfMass=[0 0 0]  CenterOfMassUnits=m  MomentsOfInertia=[1 1 1]  MomentsOfInertiaUnits=kg*m^2  ProductsOfInertia=[0 0 0]  ProductsOfInertiaUnits=kg*m^2  DensityBased=off  Density=1000  DensityUnits=kg/(m^3)  DoExposeReferenceFrame=on  SerializedFrames=<Frames/>  GraphicType=FromGeometry  MarkerShape=Sphere  MarkerSize=10  MarkerSizeUnits=m  GraphicVisPropType=SimpleVisualProperties  GraphicDiffuseColor=[0.0 0.0 0.8]  GraphicSpecularColor=[0.5 0.5 0.5 1.0]  GraphicAmbientColor=[0.15 0.15 0.15 1.0]  GraphicEmissiveColor=[0.0 0.0 0.0 1.0]  GraphicShininess=100  GraphicOpacity=1.0  GeometryShape=Brick  RectangleSize=[1 1]  RectangleSizeUnits=m  BrickDimensions=[0.9 0.001 0.001]  BrickDimensionUnits=m  CylinderRadius=0.02  CylinderRadiusUnits=m  CylinderLength=1  CylinderLengthUnits=m  SphereRadius=1  SphereRadiusUnits=m  EllipsoidRadii=[1 1 1]  EllipsoidRadiiUnits=m  ExtrusionCrossSection=[1 1; -1 1; -1 -1; 1 -1]  ExtrusionCrossSectionUnits=m  ExtrusionLength=1  ExtrusionLengthUnits=m  PolygonNumSides=3  PolygonOuterRadius=1  PolygonOuterRadiusUnits=m  ExtGeomFileType=STL  ExtGeomFileUnits=m  RevolutionCrossSection=[1 1; 1 -1; 2 -1; 2 1]  RevolutionCrossSectionUnits=m  RevolutionExtent=Full  RevolutionAngle=180  RevolutionAngleUnits=deg
  "betl2 " : sm_lib/Body Elements/Solid  InertiaType=PointMass  Mass=0  MassUnits=kg  CenterOfMass=[0 0 0]  CenterOfMassUnits=m  MomentsOfInertia=[1 1 1]  MomentsOfInertiaUnits=kg*m^2  ProductsOfInertia=[0 0 0]  ProductsOfInertiaUnits=kg*m^2  DensityBased=off  Density=1000  DensityUnits=kg/(m^3)  DoExposeReferenceFrame=on  SerializedFrames=<Frames/>  GraphicType=FromGeometry  MarkerShape=Sphere  MarkerSize=10  MarkerSizeUnits=m  GraphicVisPropType=SimpleVisualProperties  GraphicDiffuseColor=[0.0 0.0 0.8]  GraphicSpecularColor=[0.5 0.5 0.5 1.0]  GraphicAmbientColor=[0.15 0.15 0.15 1.0]  GraphicEmissiveColor=[0.0 0.0 0.0 1.0]  GraphicShininess=100  GraphicOpacity=1.0  GeometryShape=Brick  RectangleSize=[1 1]  RectangleSizeUnits=m  BrickDimensions=[0.9 0.001 0.001]  BrickDimensionUnits=m  CylinderRadius=0.02  CylinderRadiusUnits=m  CylinderLength=1  CylinderLengthUnits=m  SphereRadius=1  SphereRadiusUnits=m  EllipsoidRadii=[1 1 1]  EllipsoidRadiiUnits=m  ExtrusionCrossSection=[1 1; -1 1; -1 -1; 1 -1]  ExtrusionCrossSectionUnits=m  ExtrusionLength=1  ExtrusionLengthUnits=m  PolygonNumSides=3  PolygonOuterRadius=1  PolygonOuterRadiusUnits=m  ExtGeomFileType=STL  ExtGeomFileUnits=m  RevolutionCrossSection=[1 1; 1 -1; 2 -1; 2 1]  RevolutionCrossSectionUnits=m  RevolutionExtent=Full  RevolutionAngle=180  RevolutionAngleUnits=deg
  Conn1 : PMIOPort  Port=1  Side=Right
  connections:
  Rigid Transform19/RConn1 -- Rigid Transform15/LConn1
  Rigid Transform14/LConn1 -- Rigid Transform15/RConn1 -- belt/RConn1
  Rigid Transform14/RConn1 -- "betl2 "/RConn1
  Rigid Transform19/LConn1 -- Conn1/RConn1

== system Simscape_crane_software_model/Crane1/Frame/XBelts1 ==
  Rigid Transform14 : sm_lib/Frames and Transforms/Rigid Transform  TranslationMethod=StandardAxis  TranslationStandardOffset=0.06  TranslationLengthUnit=m  TranslationStandardAxis=-Z  TranslationCartesianOffset="[-0.5 0  0]"  TranslationROffset=0  TranslationROffsetUnits=m  TranslationZOffset=0  TranslationZOffsetUnits=m  TranslationThetaOffset=0  TranslationThetaOffsetUnits=deg  RotationMethod=None  RotationAngleUnits=deg  RotationStandardAxis=+Y  RotationAngle=90  RotationArbitraryAxis=[0 0 1]  FollAlignAxisA=+X  BaseAlignAxisA=+Y  FollAlignAxisB=+Y  BaseAlignAxisB=+Z  RotationSequenceAxes=FollowerAxes  RotationSequence=XYX  RotationSequenceAngles=[0 0 0]  RotationSequenceAnglesUnits=deg  RotationMatrix=[1 0 0; 0 1 0; 0 0 1]
  Rigid Transform15 : sm_lib/Frames and Transforms/Rigid Transform  TranslationMethod=StandardAxis  TranslationStandardOffset=0.02  TranslationLengthUnit=m  TranslationStandardAxis=+Z  TranslationCartesianOffset="[-0.5 0  0]"  TranslationROffset=0  TranslationROffsetUnits=m  TranslationZOffset=0  TranslationZOffsetUnits=m  TranslationThetaOffset=0  TranslationThetaOffsetUnits=deg  RotationMethod=None  RotationAngleUnits=deg  RotationStandardAxis=+Y  RotationAngle=90  RotationArbitraryAxis=[0 0 1]  FollAlignAxisA=+X  BaseAlignAxisA=+Y  FollAlignAxisB=+Y  BaseAlignAxisB=+Z  RotationSequenceAxes=FollowerAxes  RotationSequence=XYX  RotationSequenceAngles=[0 0 0]  RotationSequenceAnglesUnits=deg  RotationMatrix=[1 0 0; 0 1 0; 0 0 1]
  Rigid Transform19 : sm_lib/Frames and Transforms/Rigid Transform  TranslationMethod=StandardAxis  TranslationStandardOffset=0.43  TranslationLengthUnit=m  TranslationStandardAxis=-X  TranslationCartesianOffset="[-0.5 0  0]"  TranslationROffset=0  TranslationROffsetUnits=m  TranslationZOffset=0  TranslationZOffsetUnits=m  TranslationThetaOffset=0  TranslationThetaOffsetUnits=deg  RotationMethod=None  RotationAngleUnits=deg  RotationStandardAxis=+Y  RotationAngle=90  RotationArbitraryAxis=[0 0 1]  FollAlignAxisA=+X  BaseAlignAxisA=+Y  FollAlignAxisB=+Y  BaseAlignAxisB=+Z  RotationSequenceAxes=FollowerAxes  RotationSequence=XYX  RotationSequenceAngles=[0 0 0]  RotationSequenceAnglesUnits=deg  RotationMatrix=[1 0 0; 0 1 0; 0 0 1]
  belt : sm_lib/Body Elements/Solid  InertiaType=PointMass  Mass=0  MassUnits=kg  CenterOfMass=[0 0 0]  CenterOfMassUnits=m  MomentsOfInertia=[1 1 1]  MomentsOfInertiaUnits=kg*m^2  ProductsOfInertia=[0 0 0]  ProductsOfInertiaUnits=kg*m^2  DensityBased=off  Density=1000  DensityUnits=kg/(m^3)  DoExposeReferenceFrame=on  SerializedFrames=<Frames/>  GraphicType=FromGeometry  MarkerShape=Sphere  MarkerSize=10  MarkerSizeUnits=m  GraphicVisPropType=SimpleVisualProperties  GraphicDiffuseColor=[0.0 0.0 0.8]  GraphicSpecularColor=[0.5 0.5 0.5 1.0]  GraphicAmbientColor=[0.15 0.15 0.15 1.0]  GraphicEmissiveColor=[0.0 0.0 0.0 1.0]  GraphicShininess=100  GraphicOpacity=1.0  GeometryShape=Brick  RectangleSize=[1 1]  RectangleSizeUnits=m  BrickDimensions=[0.9 0.001 0.001]  BrickDimensionUnits=m  CylinderRadius=0.02  CylinderRadiusUnits=m  CylinderLength=1  CylinderLengthUnits=m  SphereRadius=1  SphereRadiusUnits=m  EllipsoidRadii=[1 1 1]  EllipsoidRadiiUnits=m  ExtrusionCrossSection=[1 1; -1 1; -1 -1; 1 -1]  ExtrusionCrossSectionUnits=m  ExtrusionLength=1  ExtrusionLengthUnits=m  PolygonNumSides=3  PolygonOuterRadius=1  PolygonOuterRadiusUnits=m  ExtGeomFileType=STL  ExtGeomFileUnits=m  RevolutionCrossSection=[1 1; 1 -1; 2 -1; 2 1]  RevolutionCrossSectionUnits=m  RevolutionExtent=Full  RevolutionAngle=180  RevolutionAngleUnits=deg
  "betl2 " : sm_lib/Body Elements/Solid  InertiaType=PointMass  Mass=0  MassUnits=kg  CenterOfMass=[0 0 0]  CenterOfMassUnits=m  MomentsOfInertia=[1 1 1]  MomentsOfInertiaUnits=kg*m^2  ProductsOfInertia=[0 0 0]  ProductsOfInertiaUnits=kg*m^2  DensityBased=off  Density=1000  DensityUnits=kg/(m^3)  DoExposeReferenceFrame=on  SerializedFrames=<Frames/>  GraphicType=FromGeometry  MarkerShape=Sphere  MarkerSize=10  MarkerSizeUnits=m  GraphicVisPropType=SimpleVisualProperties  GraphicDiffuseColor=[0.0 0.0 0.8]  GraphicSpecularColor=[0.5 0.5 0.5 1.0]  GraphicAmbientColor=[0.15 0.15 0.15 1.0]  GraphicEmissiveColor=[0.0 0.0 0.0 1.0]  GraphicShininess=100  GraphicOpacity=1.0  GeometryShape=Brick  RectangleSize=[1 1]  RectangleSizeUnits=m  BrickDimensions=[0.9 0.001 0.001]  BrickDimensionUnits=m  CylinderRadius=0.02  CylinderRadiusUnits=m  CylinderLength=1  CylinderLengthUnits=m  SphereRadius=1  SphereRadiusUnits=m  EllipsoidRadii=[1 1 1]  EllipsoidRadiiUnits=m  ExtrusionCrossSection=[1 1; -1 1; -1 -1; 1 -1]  ExtrusionCrossSectionUnits=m  ExtrusionLength=1  ExtrusionLengthUnits=m  PolygonNumSides=3  PolygonOuterRadius=1  PolygonOuterRadiusUnits=m  ExtGeomFileType=STL  ExtGeomFileUnits=m  RevolutionCrossSection=[1 1; 1 -1; 2 -1; 2 1]  RevolutionCrossSectionUnits=m  RevolutionExtent=Full  RevolutionAngle=180  RevolutionAngleUnits=deg
  Conn1 : PMIOPort  Port=1  Side=Right
  connections:
  Rigid Transform19/LConn1 -- Conn1/RConn1
  Rigid Transform14/RConn1 -- "betl2 "/RConn1
  Rigid Transform15/RConn1 -- belt/RConn1 -- Rigid Transform14/LConn1
  Rigid Transform19/RConn1 -- Rigid Transform15/LConn1

== system Simscape_crane_software_model/Crane1/Frame/XMotorAesthetics ==
  Motor : Subsystem
  Rigid Transform13 : sm_lib/Frames and Transforms/Rigid Transform  TranslationMethod=StandardAxis  TranslationStandardOffset=0.03  TranslationLengthUnit=m  TranslationStandardAxis=-Y  TranslationCartesianOffset=[-0.5 -0.5 1]  TranslationROffset=0  TranslationROffsetUnits=m  TranslationZOffset=0  TranslationZOffsetUnits=m  TranslationThetaOffset=0  TranslationThetaOffsetUnits=deg  RotationMethod=None  RotationAngleUnits=deg  RotationStandardAxis=+X  RotationAngle=90  RotationArbitraryAxis=[0 0 1]  FollAlignAxisA=+X  BaseAlignAxisA=+Y  FollAlignAxisB=+Y  BaseAlignAxisB=+Z  RotationSequenceAxes=FollowerAxes  RotationSequence=XYX  RotationSequenceAngles=[0 0 0]  RotationSequenceAnglesUnits=deg  RotationMatrix=[1 0 0; 0 1 0; 0 0 1]
  Rigid Transform16 : sm_lib/Frames and Transforms/Rigid Transform  TranslationMethod=StandardAxis  TranslationStandardOffset=0.08  TranslationLengthUnit=m  TranslationStandardAxis=-Y  TranslationCartesianOffset=[-0.5 -0.5 1]  TranslationROffset=0  TranslationROffsetUnits=m  TranslationZOffset=0  TranslationZOffsetUnits=m  TranslationThetaOffset=0  TranslationThetaOffsetUnits=deg  RotationMethod=None  RotationAngleUnits=deg  RotationStandardAxis=+X  RotationAngle=90  RotationArbitraryAxis=[0 0 1]  FollAlignAxisA=+X  BaseAlignAxisA=+Y  FollAlignAxisB=+Y  BaseAlignAxisB=+Z  RotationSequenceAxes=FollowerAxes  RotationSequence=XYX  RotationSequenceAngles=[0 0 0]  RotationSequenceAnglesUnits=deg  RotationMatrix=[1 0 0; 0 1 0; 0 0 1]
  Rigid Transform18 : sm_lib/Frames and Transforms/Rigid Transform  TranslationMethod=None  TranslationStandardOffset=0.04  TranslationLengthUnit=m  TranslationStandardAxis=-Y  TranslationCartesianOffset=[-0.5 -0.5 1]  TranslationROffset=0  TranslationROffsetUnits=m  TranslationZOffset=0  TranslationZOffsetUnits=m  TranslationThetaOffset=0  TranslationThetaOffsetUnits=deg  RotationMethod=StandardAxis  RotationAngleUnits=deg  RotationStandardAxis=+X  RotationAngle=90  RotationArbitraryAxis=[0 0 1]  FollAlignAxisA=+X  BaseAlignAxisA=+Y  FollAlignAxisB=+Y  BaseAlignAxisB=+Z  RotationSequenceAxes=FollowerAxes  RotationSequence=XYX  RotationSequenceAngles=[0 0 0]  RotationSequenceAnglesUnits=deg  RotationMatrix=[1 0 0; 0 1 0; 0 0 1]
  Solid3 : sm_lib/Body Elements/Solid  InertiaType=PointMass  Mass=0  MassUnits=kg  CenterOfMass=[0 0 0]  CenterOfMassUnits=m  MomentsOfInertia=[1 1 1]  MomentsOfInertiaUnits=kg*m^2  ProductsOfInertia=[0 0 0]  ProductsOfInertiaUnits=kg*m^2  DensityBased=off  Density=0  DensityUnits=kg/(m^3)  DoExposeReferenceFrame=on  SerializedFrames=<Frames/>  GraphicType=FromGeometry  MarkerShape=Sphere  MarkerSize=10  MarkerSizeUnits=m  GraphicVisPropType=SimpleVisualProperties  GraphicDiffuseColor=[0.6 0.6 0.6]  GraphicSpecularColor=[0.5 0.5 0.5 1.0]  GraphicAmbientColor=[0.15 0.15 0.15 1.0]  GraphicEmissiveColor=[0.0 0.0 0.0 1.0]  GraphicShininess=75  GraphicOpacity=1  GeometryShape=Cylinder  RectangleSize=[1 1]  RectangleSizeUnits=m  BrickDimensions=[0.15 0.02 0.15]  BrickDimensionUnits=m  CylinderRadius=0.015  CylinderRadiusUnits=m  CylinderLength=0.07  CylinderLengthUnits=m  SphereRadius=1  SphereRadiusUnits=m  EllipsoidRadii=[1 1 1]  EllipsoidRadiiUnits=m  ExtrusionCrossSection=[1 1; -1 1; -1 -1; 1 -1]  ExtrusionCrossSectionUnits=m  ExtrusionLength=1  ExtrusionLengthUnits=m  PolygonNumSides=3  PolygonOuterRadius=1  PolygonOuterRadiusUnits=m  ExtGeomFileType=STL  ExtGeomFileUnits=m  RevolutionCrossSection=[1 1; 1 -1; 2 -1; 2 1]  RevolutionCrossSectionUnits=m  RevolutionExtent=Full  RevolutionAngle=180  RevolutionAngleUnits=deg
  Conn1 : PMIOPort  Port=1  Side=Left
  connections:
  Rigid Transform13/LConn1 -- Conn1/RConn1
  Motor/LConn1 -- Rigid Transform16/RConn1
  Rigid Transform16/LConn1 -- Rigid Transform18/LConn1 -- Rigid Transform13/RConn1
  Rigid Transform18/RConn1 -- Solid3/RConn1
